simulink model "gardner_vfracdelay"  (Simulink 6.0)
settings: Solver=FixedStepDiscrete  SolverMode=SingleTasking  StartTime=0.0  StopTime=tsym*(numSymb*R-1)  RelTol=1e-3
PreLoadFcn:
  | L = 16; M = 8; tsym = 0.01; numSymb = 200; snrdB = 40;
  | R = 10; rollOff = 0.75; filtDelay = 3; g = 0.07;
StartFcn:
  | if (exist('h') & ishandle(h))
  |    close(h);
  | end
StopFcn:
  | a = squeeze(delay).'; b = a(ones(numSymb,1), :); b = b(:);
  | h = figure; set(gcf,'position', [452 104 473 342]);
  | plot(b, 'b'); hold on; pause(1);plot(tau_fb,'r'); grid on; xlabel('Symbols');
  | ylabel('in Samples Per Symbol'); title('Delay Estimates');
  | legend('Actual','Estimated');
undefined symbols (not defined in the file or in its folder): randint, slcm
libraries: commsink2 x2, commdigbbndpm2 x2, commfilt2 x2, commchan2 x1, commtimrec2 x1, commrandsrc2 x1, dspsrcs4 x1, dspsigops x1
CloseFcn:
  | % clear figure handle
  | if exist('h')
  | if ishandle(h)
  |    close(h);
  | end
  | end
  | 
  | % Clear model parameters
  | clear L R g rollOff tsym M filtDelay numSymb snrdB a b g tau_fb delay h
  | 
  | % Clear signal logging variable
  | clear gardnerSigsOut
settings Model: Creator=akansal  LastModifiedBy=arodrigu  ExtModeAutoUpdateStatusClock=off  ProdHWDeviceType=Specified
settings DataIOCC: SaveOutput=off  SaveTime=off  SignalLoggingName=gardnerSigsOut
settings DebuggingCC: CheckExecutionContextPreStartOutputMsg=on  CheckExecutionContextRuntimeOutputMsg=on  SolverPrmCheckMsg=none  InheritedTsInSrcMsg=none
settings HardwareCC: ProdHWDeviceType=Specified
settings ModelReferenceCC: UpdateModelReferenceTargets=IfOutOfDate
settings CodeAppCC: MangleLength=5

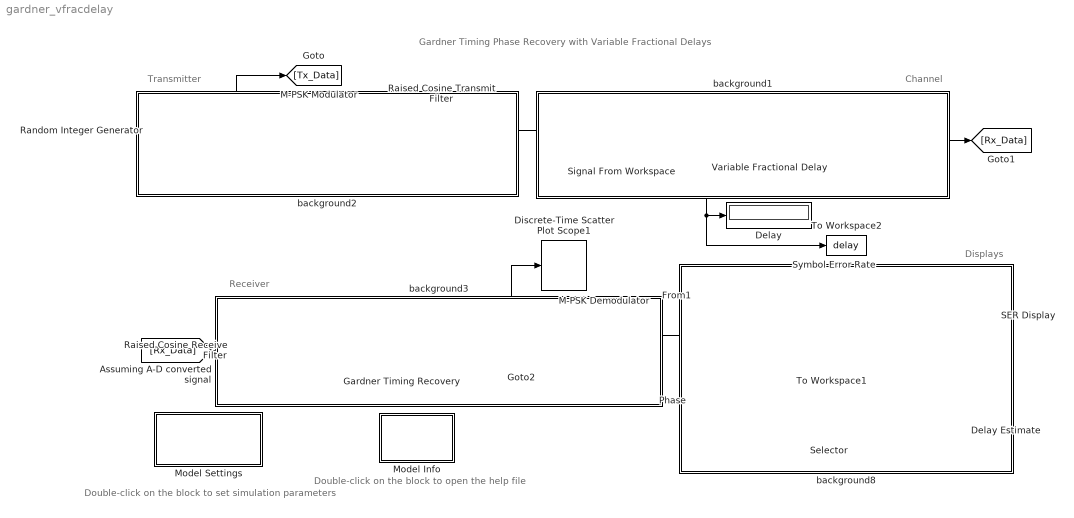
== system gardner_vfracdelay ==
  note: Gardner Timing Phase Recovery
      | with Variable Fractional Delays
  note: Channel
  note: Transmitter
  note: Receiver
  note: Displays
  note: Double-click on the block
      | to set simulation parameters
  note: Double-click on the block
      | to open the help file
  " " : commchan2/AWGN Channel  seed=61  noiseMode="Signal to noise ratio  (SNR)"  EbNodB=10  EsNodB=snrdB + 10*log10(L)  SNRdB=snrdB  bitsPerSym=1  Ps=1  Tsym=tsym  variance=0.0
  Delay : Display
  Delay Estimate : Display
  Discrete-Time Scatter Plot Scope1 : commsink2/Discrete-Time Scatter Plot Scope  Tag=ScatterPlot  sampPerSymb=1  offsetEye=0  numTraces=40  numNewFrames=10  LineMarkers=*  LineColors=b  fading=off  render=off  AxisGrid=on  xMin=-1.19037466930143  xMax=1.17408434358489  yMin=-1.17688403841458  yMax=1.18757497447174  inphaseLabel=In-phase Amplitude  quadratureLabel=Quadrature Amplitude  openScopeAtSimStart=on  FrameNumber=off  FigPos=[67 96 375 375]  figTitle=Rx Symbols  numLinesMax=8  block_type_=scatter
  Gardner Timing Recovery : commtimrec2/Gardner Timing Recovery  sampPerSymbol=L  propGain=g  resetMode=None
  M-PSK Demodulator : commdigbbndpm2/M-PSK Demodulator Baseband  M=M  OutType=Integer  Dec=Binary  Ph=0  numSamp=1
  M-PSK Modulator : commdigbbndpm2/M-PSK Modulator Baseband  M=M  InType=Integer  Enc=Binary  Ph=0  numSamp=1
  Model Info : Subsystem  LoadFcn=slcm LoadBlock;  InitFcn=slcm('UpdateAllCMBlocksInThisModelInit')  PropExecContextAcrossSSBoundary=on  mask(CMBlock){InitialSaveTempField=, InitialBlockCM=None, BlockCM=None, Frame=on, SaveTempField=, DisplayStringWithTags=Info, MaskDisplayString=Info, HorizontalTextAlignment=Center, LeftAlignmentValue=0.5, SourceBlockDiagram=gardner_vfracdelay, TagMaxNumber=20, CMTag1=, CMTag2=, CMTag3=, CMTag4=, CMTag5=, CMTag6=, CMTag7=, CMTag8=, CMTag9=, CMTag10=, CMTag11=, CMTag12=, CMTag13=, CMTag14=, CMTag15=, CMTag16=, CMTag17=, CMTag18=, CMTag19=, CMTag20=}
      mask help: This block allows revision control information to be displayed within the model.
      settings: CopyFcn=slcm CopyBlock;  DeleteFcn=slcm Cancel;  PostSaveFcn=slcm('UpdateAllCMBlocksInThisModel')  NameChangeFcn=slcm Rename;  OpenFcn=commdemohelp;
      mask Display: text(str2num(LeftAlignmentValue), 0.5, MaskDisplayString, 'HorizontalAlignment', HorizontalTextAlignment)
  Model Settings : Subsystem  PropExecContextAcrossSSBoundary=on  mask(Initial Model Settings){M=8, tsym=0.01, g=0.07, snrdB=30, L=16, rollOff=0.75, filtDelay=3, numSymb=100, numRuns=25}
      mask prompts: M "Alphabet size (M):"; tsym "Symbol period:"; g "Step size (g):"; snrdB "SNR (dB):"; L "Oversampling factor (L):"; rollOff "Rolloff factor:"; filtDelay "Group Delay:"; numSymb "Number of symbols per frame:"; numRuns "Number of frames:"
      mask help: Sets the different parameters for a simulation run.
      mask init:
      | gardner_masksetup(gcb);
      mask Display: disp('Initial Model\nSettings');
  Raised Cosine Receive Filter : commfilt2/Raised Cosine Receive Filter  filtType=Square root  N=L  D=filtDelay  R=rollOff  sampMode=Frame-based  rateMode=None  downFactor=1  downOffset=0  checkGain=Normalized  filterGain=1  checkCoeff=off  variableName=rcRxFilt  launchFVT=off
  Raised Cosine Transmit Filter : commfilt2/Raised Cosine Transmit Filter  filtType=Square root  D=filtDelay  R=rollOff  sampMode=Frame-based  N=L  checkGain=Normalized  filterGain=1  checkCoeff=off  variableName=rcTxFilt  launchFVT=off
  Random Integer Generator : commrandsrc2/Random Integer Generator  mul=M  seed=37  Ts=tsym  frameBased=on  sampPerFrame=numSymb  orient=off
  SER Display : Display
  Selector : Selector  Elements=numSymb  InputPortWidth=numSymb
  Signal From Workspace : dspsrcs4/Signal From Workspace  X=randint(R,1,L,918) + rand(R,1)  Ts=tsym*numSymb  nsamps=1  OutputAfterFinalValue=Cyclic repetition
  Symbol Error Rate : commsink2/Error Rate Calculation  N=2*filtDelay+2  st_delay=0  cp_mode=Entire frame  subframe=[]  PMode=Port  WsName=ErrorVec  RsMode2=off  stop=off  numErr=inf  maxBits=inf
  To Workspace1 : ToWorkspace  VariableName=tau_fb  SampleTime=-1  SaveFormat=Array
  To Workspace2 : ToWorkspace  VariableName=delay  SampleTime=-1  SaveFormat=Array
  Variable Fractional Delay : dspsigops/Variable Fractional Delay  mode=Linear Interpolation  dmax=L  L=4  R=10  alpha=1  ic=0
  background1 : Subsystem  PropExecContextAcrossSSBoundary=on
      mask Display: disp('')
  background2 : Subsystem  PropExecContextAcrossSSBoundary=on
      mask Display: disp('')
  background3 : Subsystem  PropExecContextAcrossSSBoundary=on
      mask Display: disp('')
  background8 : Subsystem  PropExecContextAcrossSSBoundary=on
      mask Display: disp('')
  wires:
  M-PSK Modulator/1 -> Raised Cosine Transmit Filter/1
  Raised Cosine Transmit Filter/1 -> Variable Fractional Delay/1
  Random Integer Generator/1 -> [Tx_Data], M-PSK Modulator/1
  Symbol Error Rate/1 -> SER Display/1
  M-PSK Demodulator/1 -> Symbol Error Rate/2
  [Tx_Data] -> Symbol Error Rate/1
  [Rx_Data] -> Raised Cosine Receive Filter/1
  Selector/1 -> Delay Estimate/1
  Variable Fractional Delay/1 -> " "/1
  Gardner Timing Recovery/1 -> M-PSK Demodulator/1, Discrete-Time Scatter Plot Scope1/1
  " "/1 -> [Rx_Data]
  Signal From Workspace/1 -> Variable Fractional Delay/2, Delay/1, To Workspace2/1
  Gardner Timing Recovery/2 -> [Est_Ph]
  [Est_Ph] -> To Workspace1/1, Selector/1
  Raised Cosine Receive Filter/1 -> Gardner Timing Recovery/1

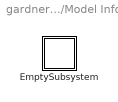
== system gardner_vfracdelay/Model Info ==
  EmptySubsystem : Subsystem  PropExecContextAcrossSSBoundary=on

== system gardner_vfracdelay/Model Settings ==

== system gardner_vfracdelay/background1 ==

== system gardner_vfracdelay/background2 ==

== system gardner_vfracdelay/background3 ==

== system gardner_vfracdelay/background8 ==

== system gardner_vfracdelay/Model Info/EmptySubsystem ==
